simulink model "CASHEW_old"  (R2023a)
settings: Solver=ode23t  StartTime=0.0  StopTime=10.0  RelTol=1e-3
libraries: fl_lib x25, nesl_utility x9, SimscapeFluids_lib x7
settings Model: Creator=degoe  LastModifiedBy=cpoki

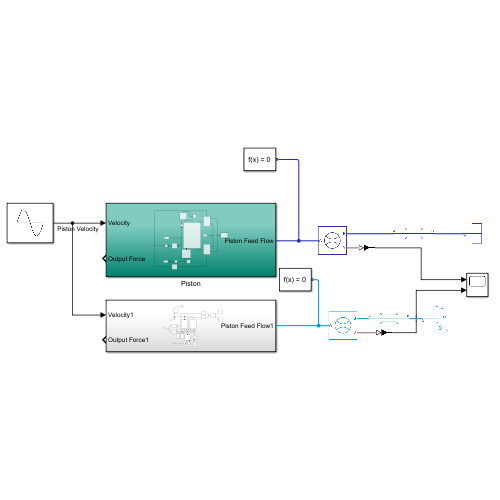
[thumbnail: Simulink's stored preview of the top-level diagram]
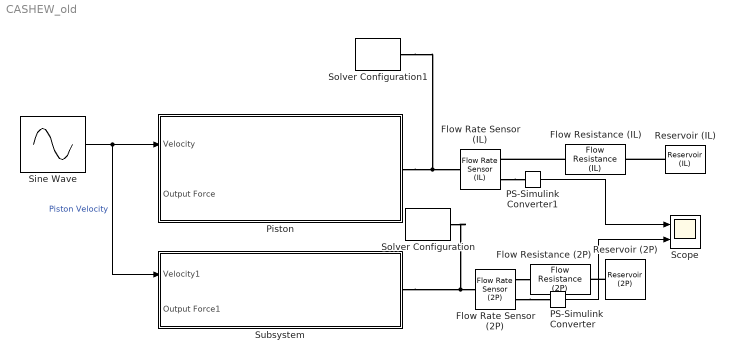
== system CASHEW_old ==
  Flow Rate Sensor (2P) : fl_lib/Two-Phase Fluid/Sensors/Flow Rate Sensor (2P)  mass_flow_measure=false  volumetric_flow_measure=true  energy_flow_measure=false
      settings: InternalSimscapePortConfiguration="{\"Bottom\":[],\"Left\":[{\"id\":\"A\",\"label\":\"A\",\"type\":\"foundation.two_phase_fluid.two_phase_fluid\"}],\"Right\":[{\"id\":\"B\",\"label\":\"B\",\"type\":\"foundation.two_phase_fluid.two_phase_fluid\"},{\"id\":\"V\",\"label\":\"V\",\"type\":\"output\"}],\"Top\":[]}"
  Flow Rate Sensor (IL) : fl_lib/Isothermal Liquid/Sensors/Flow Rate Sensor (IL)  sensor_type=foundation.enum.mass_volumetric_sensor.volumetric
      settings: InternalSimscapePortConfiguration="{\"Bottom\":[],\"Left\":[{\"id\":\"A\",\"label\":\"A\",\"type\":\"foundation.isothermal_liquid.isothermal_liquid\"}],\"Right\":[{\"id\":\"B\",\"label\":\"B\",\"type\":\"foundation.isothermal_liquid.isothermal_liquid\"},{\"id\":\"V\",\"label\":\"V\",\"type\":\"output\"}],\"Top\":[]}"
  Flow Resistance (2P) : fl_lib/Two-Phase Fluid/Elements/Flow Resistance (2P)  delta_p_nominal=0.001 MPa  mdot_nominal=0.1 kg/s  v_nominal=0 m^3/kg  area=0.01 m^2  laminar_fraction=1e-3
      settings: InternalSimscapePortConfiguration="{\"Bottom\":[],\"Left\":[{\"id\":\"A\",\"label\":\"A\",\"type\":\"foundation.two_phase_fluid.two_phase_fluid\"}],\"Right\":[{\"id\":\"B\",\"label\":\"B\",\"type\":\"foundation.two_phase_fluid.two_phase_fluid\"}],\"Top\":[]}"
  Flow Resistance (IL) : fl_lib/Isothermal Liquid/Elements/Flow Resistance (IL)  delta_p_nominal=0.001 MPa  mdot_nominal=0.1 kg/s  laminar_fraction=1e-3
      settings: InternalSimscapePortConfiguration="{\"Bottom\":[],\"Left\":[{\"id\":\"A\",\"label\":\"A\",\"type\":\"foundation.isothermal_liquid.isothermal_liquid\"}],\"Right\":[{\"id\":\"B\",\"label\":\"B\",\"type\":\"foundation.isothermal_liquid.isothermal_liquid\"}],\"Top\":[]}"
  PS-Simulink Converter : nesl_utility/PS-Simulink Converter  PhysicalDomain=network_engine_domain  SubClassName=ps_output  LeftPortType=input  RightPortType=output  PseudoPeriodic=off  Frequencies=[]  VectorFormat=inherit  Unit=inherit  AffineConversion=off
  PS-Simulink Converter1 : nesl_utility/PS-Simulink Converter  PhysicalDomain=network_engine_domain  SubClassName=ps_output  LeftPortType=input  RightPortType=output  PseudoPeriodic=off  Frequencies=[]  VectorFormat=inherit  Unit=inherit  AffineConversion=off
  Piston : Subsystem
      settings: PortSchema="{\"entries\":[{\"content\":{\"sides\":[{\"content\":{\"connectorIds\":[\"In1\",\"Out1\"]},\"type\":\"ConnectorPlacement.EquallySpacedRectSide\",\"uuid\":\"b8e78877-c290-4656-932c-79ee659867db\"},{\"content\":{\"connectorIds\":[\"RConn1\"],\"side\":\"RIGHT\"},\"type\":\"ConnectorPlacement.EquallySpacedRectSide\",\"uuid\":\"f3ba2138-776c-4b7b-9f4c-235aea75c0ff\"},{\"content\":{\"side\":\"TOP\"},\"type\":\"ConnectorPlacement.EquallySpacedRectSide\",\"uuid\":\"3b9ee6c7-725d-42d9-8cef-d327921b75c9\"}]},\"type\":\"ConnectorPlacement.EquallySpacedConnector\",\"uuid\":\"ca70cb4f-6465-4ac9-9ae0-4b805d4678c7\"}],\"packageUris\":[\"http://schema.mathworks.com/mf0/Connector/R2020b\"],\"version\":\"1.0\"}"
  Reservoir (2P) : fl_lib/Two-Phase Fluid/Elements/Reservoir (2P)  pressure_spec=foundation.enum.ReservoirPressureSpec2P.Atmospheric  reservoir_pressure=0.101325 MPa  reservoir_condensing_temperature=373.15 K  reservoir_evaporating_temperature=373.15 K  energy_spec=foundation.enum.ReservoirEnergySpec2P.Temperature  reservoir_temperature=293.15 K  reservoir_quality=0.5  reservoir_void_fraction=0.5  reservoir_enthalpy=1500 kJ/kg  reservoir_internal_energy=1500 kJ/kg  reservoir_subcooling=5 deltaK  reservoir_superheating=5 deltaK  area_A=0.01 m^2
  Reservoir (IL) : fl_lib/Isothermal Liquid/Elements/Reservoir (IL)  reservoir_type=foundation.enum.constant_controlled.constant  pressure_spec=foundation.enum.pressure_spec.atmospheric  reservoir_pressure=0.101325 MPa
  Scope : Scope  NumInputPorts=2
  Sine Wave : Sin  Amplitude=0.37233113  Frequency=0.7  SampleTime=0
  Solver Configuration : nesl_utility/Solver Configuration  PhysicalDomain=network_engine_domain  SubClassName=solver  LeftPortType=input  RightPortType=generic  Tones=[]  Harmonics=[]  SimulateNoise=off  Profile=off  UseLocalSampling=off  EnableSwitchedLinearOptims=on  FrequencyDomain=off  UseCCode=off  RelTol=0.001  AbsTol=0.001  MinStep=1e-09  ToWorkspace=off  RevertToSquareIcSolve=off  NumHomotopyIterations=100  PhasorMode=off  PhasorModeNumHarmonics=1  ConsistencySolver=NEWTON_XTOL_AFTER_FTOL  IndexReductionMethod=DerivativeReplacement  DoDC=off  ResidualTolerance=1e-09  ConsistencyTolSource=GLOBAL  ConsistencyAbsTol=0.001  ConsistencyRelTol=0.001  ConsistencyTolFactor=0.001  UseLocalSolver=off  LocalSolverChoice=NE_BACKWARD_EULER_ADVANCER  ResolveIndetEquations=on  FunctionEvalNumThread=1  LocalSolverSampleTime=0.001  DoFixedCost=off  MaxNonlinIter=3  MaxModeIter=2  ComputeImpulses=off  ImpulseIterations=2  LinearAlgebra=auto  LinearAlgebraNumThread=0  EquationFormulation=NE_TIME_EF  DelaysMemoryBudget=1024  AutomaticFiltering=on  FilteringTimeConstant=0.001  PartitionStorageMethod=AS_NEEDED  PartitionMemoryBudget=1024  PartitionMethod=ROBUST
  Solver Configuration1 : nesl_utility/Solver Configuration  PhysicalDomain=network_engine_domain  SubClassName=solver  LeftPortType=input  RightPortType=generic  Tones=[]  Harmonics=[]  SimulateNoise=off  Profile=off  UseLocalSampling=off  EnableSwitchedLinearOptims=on  FrequencyDomain=off  UseCCode=off  RelTol=0.001  AbsTol=0.001  MinStep=1e-09  ToWorkspace=off  RevertToSquareIcSolve=off  NumHomotopyIterations=100  PhasorMode=off  PhasorModeNumHarmonics=1  ConsistencySolver=NEWTON_XTOL_AFTER_FTOL  IndexReductionMethod=DerivativeReplacement  DoDC=off  ResidualTolerance=1e-09  ConsistencyTolSource=GLOBAL  ConsistencyAbsTol=0.001  ConsistencyRelTol=0.001  ConsistencyTolFactor=0.001  UseLocalSolver=off  LocalSolverChoice=NE_BACKWARD_EULER_ADVANCER  ResolveIndetEquations=on  FunctionEvalNumThread=1  LocalSolverSampleTime=0.001  DoFixedCost=off  MaxNonlinIter=3  MaxModeIter=2  ComputeImpulses=off  ImpulseIterations=2  LinearAlgebra=auto  LinearAlgebraNumThread=0  EquationFormulation=NE_TIME_EF  DelaysMemoryBudget=1024  AutomaticFiltering=on  FilteringTimeConstant=0.001  PartitionStorageMethod=AS_NEEDED  PartitionMemoryBudget=1024  PartitionMethod=ROBUST
  Subsystem : Subsystem
      settings: PortSchema="{\"entries\":[{\"content\":{\"sides\":[{\"content\":{\"connectorIds\":[\"In1\",\"Out1\"]},\"type\":\"ConnectorPlacement.EquallySpacedRectSide\",\"uuid\":\"3893c117-58f4-444a-acc3-3c8ad39863db\"},{\"content\":{\"connectorIds\":[\"RConn1\"],\"side\":\"RIGHT\"},\"type\":\"ConnectorPlacement.EquallySpacedRectSide\",\"uuid\":\"ce571c28-2e26-43fb-8d91-15cc15892142\"},{\"content\":{\"side\":\"TOP\"},\"type\":\"ConnectorPlacement.EquallySpacedRectSide\",\"uuid\":\"309e5996-fe42-4b39-b1f7-b2ffb0eab9ca\"}]},\"type\":\"ConnectorPlacement.EquallySpacedConnector\",\"uuid\":\"baf7f0f0-8da0-4833-91c3-445f9acfddc8\"}],\"packageUris\":[\"http://schema.mathworks.com/mf0/Connector/R2020b\"],\"version\":\"1.0\"}"
  wires:
  Sine Wave/1 -> Subsystem/1(Velocity1), Piston/1(Velocity)  "Piston Velocity"
  PS-Simulink Converter1/1 -> Scope/1
  PS-Simulink Converter/1 -> Scope/2
  connections:
  Subsystem/RConn1 -- Solver Configuration/RConn1 -- Flow Rate Sensor (2P)/LConn1
  Flow Rate Sensor (2P)/RConn1 -- Flow Resistance (2P)/LConn1
  Flow Rate Sensor (2P)/RConn2 -- PS-Simulink Converter/LConn1
  Piston/RConn1 -- Solver Configuration1/RConn1 -- Flow Rate Sensor (IL)/LConn1
  Flow Resistance (IL)/LConn1 -- Flow Rate Sensor (IL)/RConn1
  Flow Rate Sensor (IL)/RConn2 -- PS-Simulink Converter1/LConn1
  Reservoir (IL)/LConn1 -- Flow Resistance (IL)/RConn1
  Reservoir (2P)/LConn1 -- Flow Resistance (2P)/RConn1

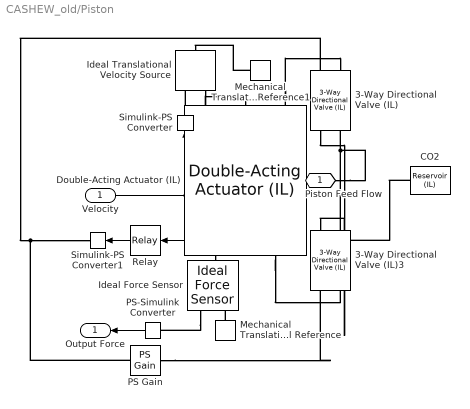
== system CASHEW_old/Piston ==
  Velocity : Inport
  3-Way Directional Valve (IL) : SimscapeFluids_lib/Isothermal Liquid/Valves & Orifices/Directional Control Valves/3-Way Directional Valve (IL)  open_orifices_pos=fluids.isothermal_liquid.valves_orifices.directional_control_valves.enum.DirectionalValveOpenOrifices3Way.PA  open_orifices_neg=fluids.isothermal_liquid.valves_orifices.directional_control_valves.enum.DirectionalValveOpenOrifices3Way.AT  area_spec=fluids.isothermal_liquid.valves_orifices.directional_control_valves.enum.directional_valve_area_spec.identical  valve_spec=fluids.isothermal_liquid.valves_orifices.directional_control_valves.enum.directional_valve_spec.linear  del_S_max=1 m  area_max=0.05 m^2  del_S_TLU=[0, .00125, .0025, .00375, .005] m  valve_area_TLU=[1e-10, 1e-05, 4e-05, 8e-05, .0001] m^2  del_S_vol_flow_TLU=[0, .00125, .0025, .00375, .005] m  p_diff_TLU=[-.1, .3, .5, .7] MPa  vol_flow_TLU=[-9.05e-10, 1.57e-09, 2.02e-09, 2.39e-09; -9.05e-05, .000157, .000202, .000239; -.000362, .000627, .00081, .000958; -.000724, .00125, .00162, .00192; -.000905, .00156, .002, .00239] m^3/s  area=inf m^2  area_leak=1e-15 m^2  Cd=0.7  Re_c=15000  smoothing_factor=0.01  pressure_recovery=false  S_max_PA=1 m  del_S_max_PA=0.005 m  area_max_PA=1e-4 m^2  del_S_TLU_PA=[0, .00125, .0025, .00375, .005] m  valve_area_TLU_PA=[1e-10, 1e-05, 4e-05, 8e-05, .0001] m^2  del_S_vol_flow_TLU_PA=[0, .00125, .0025, .00375, .005] m  p_diff_TLU_PA=[-.1, .3, .5, .7] MPa  vol_flow_TLU_PA=[-9.05e-10, 1.57e-09, 2.02e-09, 2.39e-09; -9.05e-05, .000157, .000202, .000239; -.000362, .000627, .00081, .000958; -.000724, .00125, .00162, .00192; -.000905, .00156, .002, .00239] m^3/s  S_max_AT=-1 m  del_S_max_AT=0.005 m  area_max_AT=1e-4 m^2  del_S_TLU_AT=[0, .00125, .0025, .00375, .005] m  valve_area_TLU_AT=[1e-10, 1e-05, 4e-05, 8e-05, .0001] m^2  del_S_vol_flow_TLU_AT=[0, .00125, .0025, .00375, .005] m  p_diff_TLU_AT=[-.1, .3, .5, .7] MPa  vol_flow_TLU_AT=[-9.05e-10, 1.57e-09, 2.02e-09, 2.39e-09; -9.05e-05, .000157, .000202, .000239; -.000362, .000627, .00081, .000958; -.000724, .00125, .00162, .00192; -.000905, .00156, .002, .00239] m^3/s  S_max_PT=4.5e-3 m  del_S_max_PT=0.005 m  area_max_PT=1e-4 m^2  del_S_TLU_PT=[0, .00125, .0025, .00375, .005] m  valve_area_TLU_PT=[1e-10, 1e-05, 4e-05, 8e-05, .0001] m^2  del_S_vol_flow_TLU_PT=[0, .00125, .0025, .00375, .005] m  p_diff_TLU_PT=[-.1, .3, .5, .7] MPa  vol_flow_TLU_PT=[-9.05e-10, 1.57e-09, 2.02e-09, 2.39e-09; -9.05e-05, .000157, .000202, .000239; -.000362, .000627, .00081, .000958; -.000724, .00125, .00162, .00192; -.000905, .00156, .002, .00239] m^3/s  enable_faults=simscape.enum.onoff.off  fault_type=fluids.enum.FaultSpool2Position.Positive  fault_trigger=foundation.enum.faultSpec.Temporal  fault_time=5 s
      settings: InternalSimscapePortConfiguration="{\"Bottom\":[{\"id\":\"P\",\"label\":\"P\",\"type\":\"foundation.isothermal_liquid.isothermal_liquid\"},{\"id\":\"T\",\"label\":\"T\",\"type\":\"foundation.isothermal_liquid.isothermal_liquid\"}],\"Left\":[{\"id\":\"S\",\"label\":\"S\",\"type\":\"input\"}],\"Right\":[],\"Top\":[{\"id\":\"A\",\"label\":\"A\",\"type\":\"foundation.isothermal_liquid.isothermal_liquid\"}]}"
  3-Way Directional Valve (IL)3 : SimscapeFluids_lib/Isothermal Liquid/Valves & Orifices/Directional Control Valves/3-Way Directional Valve (IL)  open_orifices_pos=fluids.isothermal_liquid.valves_orifices.directional_control_valves.enum.DirectionalValveOpenOrifices3Way.PA  open_orifices_neg=fluids.isothermal_liquid.valves_orifices.directional_control_valves.enum.DirectionalValveOpenOrifices3Way.AT  area_spec=fluids.isothermal_liquid.valves_orifices.directional_control_valves.enum.directional_valve_area_spec.identical  valve_spec=fluids.isothermal_liquid.valves_orifices.directional_control_valves.enum.directional_valve_spec.linear  del_S_max=1 m  area_max=0.05 m^2  del_S_TLU=[0, .00125, .0025, .00375, .005] m  valve_area_TLU=[1e-10, 1e-05, 4e-05, 8e-05, .0001] m^2  del_S_vol_flow_TLU=[0, .00125, .0025, .00375, .005] m  p_diff_TLU=[-.1, .3, .5, .7] MPa  vol_flow_TLU=[-9.05e-10, 1.57e-09, 2.02e-09, 2.39e-09; -9.05e-05, .000157, .000202, .000239; -.000362, .000627, .00081, .000958; -.000724, .00125, .00162, .00192; -.000905, .00156, .002, .00239] m^3/s  area=inf m^2  area_leak=1e-15 m^2  Cd=0.7  Re_c=15000  smoothing_factor=0.01  pressure_recovery=false  S_max_PA=1 m  del_S_max_PA=0.005 m  area_max_PA=1e-4 m^2  del_S_TLU_PA=[0, .00125, .0025, .00375, .005] m  valve_area_TLU_PA=[1e-10, 1e-05, 4e-05, 8e-05, .0001] m^2  del_S_vol_flow_TLU_PA=[0, .00125, .0025, .00375, .005] m  p_diff_TLU_PA=[-.1, .3, .5, .7] MPa  vol_flow_TLU_PA=[-9.05e-10, 1.57e-09, 2.02e-09, 2.39e-09; -9.05e-05, .000157, .000202, .000239; -.000362, .000627, .00081, .000958; -.000724, .00125, .00162, .00192; -.000905, .00156, .002, .00239] m^3/s  S_max_AT=-1 m  del_S_max_AT=0.005 m  area_max_AT=1e-4 m^2  del_S_TLU_AT=[0, .00125, .0025, .00375, .005] m  valve_area_TLU_AT=[1e-10, 1e-05, 4e-05, 8e-05, .0001] m^2  del_S_vol_flow_TLU_AT=[0, .00125, .0025, .00375, .005] m  p_diff_TLU_AT=[-.1, .3, .5, .7] MPa  vol_flow_TLU_AT=[-9.05e-10, 1.57e-09, 2.02e-09, 2.39e-09; -9.05e-05, .000157, .000202, .000239; -.000362, .000627, .00081, .000958; -.000724, .00125, .00162, .00192; -.000905, .00156, .002, .00239] m^3/s  S_max_PT=4.5e-3 m  del_S_max_PT=0.005 m  area_max_PT=1e-4 m^2  del_S_TLU_PT=[0, .00125, .0025, .00375, .005] m  valve_area_TLU_PT=[1e-10, 1e-05, 4e-05, 8e-05, .0001] m^2  del_S_vol_flow_TLU_PT=[0, .00125, .0025, .00375, .005] m  p_diff_TLU_PT=[-.1, .3, .5, .7] MPa  vol_flow_TLU_PT=[-9.05e-10, 1.57e-09, 2.02e-09, 2.39e-09; -9.05e-05, .000157, .000202, .000239; -.000362, .000627, .00081, .000958; -.000724, .00125, .00162, .00192; -.000905, .00156, .002, .00239] m^3/s  enable_faults=simscape.enum.onoff.off  fault_type=fluids.enum.FaultSpool2Position.Positive  fault_trigger=foundation.enum.faultSpec.Temporal  fault_time=5 s
      settings: InternalSimscapePortConfiguration="{\"Bottom\":[{\"id\":\"P\",\"label\":\"P\",\"type\":\"foundation.isothermal_liquid.isothermal_liquid\"},{\"id\":\"T\",\"label\":\"T\",\"type\":\"foundation.isothermal_liquid.isothermal_liquid\"}],\"Left\":[{\"id\":\"S\",\"label\":\"S\",\"type\":\"input\"}],\"Right\":[],\"Top\":[{\"id\":\"A\",\"label\":\"A\",\"type\":\"foundation.isothermal_liquid.isothermal_liquid\"}]}"
  CO2 : fl_lib/Isothermal Liquid/Elements/Reservoir (IL)  reservoir_type=foundation.enum.constant_controlled.constant  pressure_spec=foundation.enum.pressure_spec.atmospheric  reservoir_pressure=0.101325 MPa
  Double-Acting Actuator (IL) : SimscapeFluids_lib/Isothermal Liquid/Actuators/Double-Acting Actuator (IL)  mech_orientation=foundation.enum.MechOrientationTranslational.Positive  piston_area_A=piston_area m^2  piston_area_B=piston_area m^2  stroke=2000 m  dead_volume_A=1e-15 m^3  dead_volume_B=1e-15 m^3  pressure_spec=foundation.enum.pressure_spec.atmospheric  environment_pressure=0.101325 MPa  hardstop_model=simscape.enum.hardstop.smooth  stiff_coeff=1e10 N/m  damping_coeff=150 N*s/m  transition=0.1 mm  coeff_rest=0.7  v_tol=0.001 m/s  f_tol=0.001 N  cushion_A_spec=false  area_plunger_A=1e-4 m^2  length_plunger_A=1e-3 m  area_cushion_orifice_A=1e-6 m^2  area_leak_plunger_A=1e-7 m^2  p_crack_differential_A=0.01 MPa  press_max_differential_A=0.1 MPa  check_valve_area_max_A=1e-4 m^2  check_valve_area_leak_A=1e-10 m^2  smoothing_factor_A=0.01  cushion_B_spec=false  area_plunger_B=1e-4 m^2  length_plunger_B=1e-3 m  area_cushion_orifice_B=1e-6 m^2  area_leak_plunger_B=1e-7 m^2  p_crack_differential_B=0.01 MPa  press_max_differential_B=0.1 MPa  check_valve_area_max_B=1e-4 m^2  check_valve_area_leak_B=1e-10 m^2  smoothing_factor_B=0.01  friction_spec=false  breakaway_Coulomb_ratio=1.2  breakaway_velocity=0.1 m/s  preload_force=20 N  Coulomb_coeff=1e-6 N/Pa  viscous_coeff=100 N*s/m  leakage_spec=false  clearance=1e-4 m  piston_length=0.01 m  displacement_spec=foundation.enum.DisplacementSpec.Calculate  x0=6 m  dynamic_compressibility=false  p0_A=0.101325 MPa  p0_B=0.101325 MPa
      settings: InternalSimscapePortConfiguration="{\"Bottom\":[],\"Left\":[{\"id\":\"C\",\"label\":\"C\",\"type\":\"foundation.mechanical.translational.translational\"},{\"id\":\"A\",\"label\":\"A\",\"type\":\"foundation.isothermal_liquid.isothermal_liquid\"}],\"Right\":[{\"id\":\"p_out\",\"label\":\"p\",\"type\":\"output\"},{\"id\":\"R\",\"label\":\"R\",\"type\":\"foundation.mechanical.translational.translational\"},{\"id\":\"B\",\"label\":\"B\",\"type\":\"foundation.isothermal_liquid.isothermal_liquid\"}],\"Top\":[]}"
  Ideal Force Sensor : fl_lib/Mechanical/Mechanical Sensors/Ideal Force Sensor
  Ideal Translational Velocity Source : fl_lib/Mechanical/Mechanical Sources/Ideal Translational Velocity Source
  Mechanical Translational Reference : fl_lib/Mechanical/Translational Elements/Mechanical Translational Reference
  Mechanical Translational Reference1 : fl_lib/Mechanical/Translational Elements/Mechanical Translational Reference
  PS Gain : fl_lib/Physical Signals/Functions/PS Gain  gain=-1
  PS-Simulink Converter : nesl_utility/PS-Simulink Converter  PhysicalDomain=network_engine_domain  SubClassName=ps_output  LeftPortType=input  RightPortType=output  PseudoPeriodic=off  Frequencies=[]  VectorFormat=inherit  Unit=inherit  AffineConversion=off
  Relay : Relay  OnSwitchValue=0  OffSwitchValue=0  OffOutputValue=-1
  Simulink-PS Converter : nesl_utility/Simulink-PS Converter  PhysicalDomain=network_engine_domain  SubClassName=ps_input  LeftPortType=input  RightPortType=output  PseudoPeriodic=off  Frequencies=[]  NoiseDistribution=none  NoiseParameters=[]  Unit=m/s  AffineConversion=off  FilteringAndDerivatives=provide  SimscapeFilterOrder=1  InputFilterTimeConstant=0.001  UdotUserProvided=0
  Simulink-PS Converter1 : nesl_utility/Simulink-PS Converter  PhysicalDomain=network_engine_domain  SubClassName=ps_input  LeftPortType=input  RightPortType=output  PseudoPeriodic=off  Frequencies=[]  NoiseDistribution=none  NoiseParameters=[]  Unit=1  AffineConversion=off  FilteringAndDerivatives=provide  SimscapeFilterOrder=1  InputFilterTimeConstant=0.001  UdotUserProvided=0
  Piston Feed Flow : PMIOPort  Side=Right
  Output Force : Outport
  wires:
  Relay/1 -> Simulink-PS Converter1/1
  PS-Simulink Converter/1 -> Output Force/1
  Velocity/1 -> Simulink-PS Converter/1, Relay/1
  connections:
  PS Gain/LConn1 -- 3-Way Directional Valve (IL)/LConn1 -- Simulink-PS Converter1/RConn1
  Double-Acting Actuator (IL)/LConn1 -- Ideal Force Sensor/LConn1
  Simulink-PS Converter/RConn1 -- Ideal Translational Velocity Source/RConn1
  PS Gain/RConn1 -- 3-Way Directional Valve (IL)3/LConn1
  Double-Acting Actuator (IL)/LConn2 -- 3-Way Directional Valve (IL)3/LConn2
  Double-Acting Actuator (IL)/RConn3 -- 3-Way Directional Valve (IL)/LConn2
  3-Way Directional Valve (IL)3/RConn2 -- Piston Feed Flow/RConn1 -- 3-Way Directional Valve (IL)/RConn2
  3-Way Directional Valve (IL)/RConn1 -- CO2/LConn1 -- 3-Way Directional Valve (IL)3/RConn1
  Ideal Force Sensor/RConn2 -- PS-Simulink Converter/LConn1
  Mechanical Translational Reference/LConn1 -- Ideal Force Sensor/RConn1
  Mechanical Translational Reference1/LConn1 -- Ideal Translational Velocity Source/LConn1
  Ideal Translational Velocity Source/RConn2 -- Double-Acting Actuator (IL)/RConn2

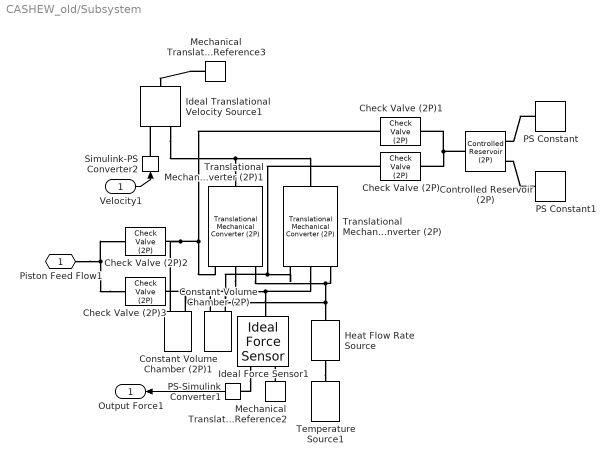
== system CASHEW_old/Subsystem ==
  Velocity1 : Inport
  Check Valve (2P){,1..3} (4 alike) : SimscapeFluids_lib/Two-Phase Fluid/Valves & Orifices/Directional Control Valves/Check Valve (2P)  opening_pressure_spec=fluids.two_phase_fluid.valves_orifices.enum.PressureControlSpec.Differential  p_crack_differential=0.01 MPa  p_crack_gauge=0.1 MPa  p_max_differential=0.1 MPa  p_max_gauge=0.2 MPa  mdot_nominal_max=0.1 kg/s  delta_p_nominal_max=0.001 MPa  energy_spec=foundation.enum.energy_spec.temperature  p_inlet=0.101325 MPa  T_inlet=293.15 K  x_inlet=0.5  alpha_inlet=0.5  h_inlet=1500 kJ/kg  u_inlet=1500 kJ/kg  area=0.01 m^2  mdot_leak_fraction=1e-6  smoothing_factor=0.01  B_lam=0.999  tau_x=0.1 s
      settings: InternalSimscapePortConfiguration="{\"Bottom\":[],\"Left\":[{\"id\":\"A\",\"label\":\"A\",\"type\":\"foundation.two_phase_fluid.two_phase_fluid\"}],\"Right\":[{\"id\":\"B\",\"label\":\"B\",\"type\":\"foundation.two_phase_fluid.two_phase_fluid\"}],\"Top\":[]}"
  Constant Volume Chamber (2P) : fl_lib/Two-Phase Fluid/Elements/Constant Volume Chamber (2P)  volume=0.001 m^3  num_ports=foundation.enum.num_ports.one  area_A=0.01 m^2  area_B=0.01 m^2  area_C=0.01 m^2  area_D=0.01 m^2  energy_spec=foundation.enum.energy_spec.temperature  p_init=0.101325 MPa  T_init=293.15 K  x_init=0.5  alpha_init=0.5  h_init=1500 kJ/kg  u_init=1500 kJ/kg  time_constant=0.1 s
      settings: InternalSimscapePortConfiguration="{\"Bottom\":[],\"Left\":[{\"id\":\"A\",\"label\":\"A\",\"type\":\"foundation.two_phase_fluid.two_phase_fluid\"},{\"id\":\"H\",\"label\":\"H\",\"type\":\"foundation.thermal.thermal\"}],\"Right\":[],\"Top\":[]}"
  Constant Volume Chamber (2P)1 : fl_lib/Two-Phase Fluid/Elements/Constant Volume Chamber (2P)  volume=0.001 m^3  num_ports=foundation.enum.num_ports.one  area_A=0.01 m^2  area_B=0.01 m^2  area_C=0.01 m^2  area_D=0.01 m^2  energy_spec=foundation.enum.energy_spec.temperature  p_init=0.101325 MPa  T_init=293.15 K  x_init=0.5  alpha_init=0.5  h_init=1500 kJ/kg  u_init=1500 kJ/kg  time_constant=0.1 s
      settings: InternalSimscapePortConfiguration="{\"Bottom\":[],\"Left\":[{\"id\":\"A\",\"label\":\"A\",\"type\":\"foundation.two_phase_fluid.two_phase_fluid\"},{\"id\":\"H\",\"label\":\"H\",\"type\":\"foundation.thermal.thermal\"}],\"Right\":[],\"Top\":[]}"
  Controlled Reservoir (2P) : fl_lib/Two-Phase Fluid/Elements/Controlled Reservoir (2P)  pressure_spec=foundation.enum.ControlledReservoirPressureSpec2P.Specified  energy_spec=foundation.enum.ControlledReservoirEnergySpec2P.LiquidTemperature  area_A=0.01 m^2  pressure_limit_spec=foundation.enum.PressureLimitSpec2P.Warn
      settings: InternalSimscapePortConfiguration="{\"Bottom\":[],\"Left\":[{\"id\":\"A\",\"label\":\"A\",\"type\":\"foundation.two_phase_fluid.two_phase_fluid\"}],\"Right\":[{\"id\":\"T\",\"label\":\"T\",\"type\":\"input\"},{\"id\":\"P\",\"label\":\"P\",\"type\":\"input\"}],\"Top\":[]}"
  Heat Flow Rate Source : fl_lib/Thermal/Thermal Sources/Heat Flow Rate Source  heat_flow=0 W
      settings: InternalSimscapePortConfiguration="{\"Bottom\":[],\"Left\":[{\"id\":\"B\",\"label\":\"B\",\"type\":\"foundation.thermal.thermal\"}],\"Right\":[{\"id\":\"A\",\"label\":\"A\",\"type\":\"foundation.thermal.thermal\"}],\"Top\":[]}"
  Ideal Force Sensor1 : fl_lib/Mechanical/Mechanical Sensors/Ideal Force Sensor
  Ideal Translational Velocity Source1 : fl_lib/Mechanical/Mechanical Sources/Ideal Translational Velocity Source
  Mechanical Translational Reference2 : fl_lib/Mechanical/Translational Elements/Mechanical Translational Reference
  Mechanical Translational Reference3 : fl_lib/Mechanical/Translational Elements/Mechanical Translational Reference
  PS Constant : fl_lib/Physical Signals/Sources/PS Constant  constant=101325 Pa
  PS Constant1 : fl_lib/Physical Signals/Sources/PS Constant  constant=293.15 K
  PS-Simulink Converter1 : nesl_utility/PS-Simulink Converter  PhysicalDomain=network_engine_domain  SubClassName=ps_output  LeftPortType=input  RightPortType=output  PseudoPeriodic=off  Frequencies=[]  VectorFormat=inherit  Unit=inherit  AffineConversion=off
  Simulink-PS Converter2 : nesl_utility/Simulink-PS Converter  PhysicalDomain=network_engine_domain  SubClassName=ps_input  LeftPortType=input  RightPortType=output  PseudoPeriodic=off  Frequencies=[]  NoiseDistribution=none  NoiseParameters=[]  Unit=m/s  AffineConversion=off  FilteringAndDerivatives=provide  SimscapeFilterOrder=1  InputFilterTimeConstant=0.001  UdotUserProvided=0
  Temperature Source1 : fl_lib/Thermal/Thermal Sources/Temperature Source  temperature=293.15 K
  Translational Mechanical Converter (2P) : fl_lib/Two-Phase Fluid/Elements/Translational Mechanical Converter (2P)  mech_orientation=foundation.enum.MechOrientationTranslational.Negative  displacement_spec=foundation.enum.DisplacementSpec.Calculate  length_init=0 m  interface_area=piston_area m^2  dead_volume=1e-5 m^3  area_A=0.01 m^2  pressure_spec=foundation.enum.pressure_spec.atmospheric  environment_pressure=0.101325 MPa  energy_spec=foundation.enum.energy_spec.temperature  p_init=0.101325 MPa  T_init=293.15 K  x_init=0.5  alpha_init=0.5  h_init=1500 kJ/kg  u_init=1500 kJ/kg  time_constant=0.1 s
      settings: InternalSimscapePortConfiguration="{\"Bottom\":[],\"Left\":[{\"id\":\"A\",\"label\":\"A\",\"type\":\"foundation.two_phase_fluid.two_phase_fluid\"},{\"id\":\"C\",\"label\":\"C\",\"type\":\"foundation.mechanical.translational.translational\"},{\"id\":\"H\",\"label\":\"H\",\"type\":\"foundation.thermal.thermal\"}],\"Right\":[{\"id\":\"R\",\"label\":\"R\",\"type\":\"foundation.mechanical.translational.translational\"}],\"Top\":[]}"
  Translational Mechanical Converter (2P)1 : fl_lib/Two-Phase Fluid/Elements/Translational Mechanical Converter (2P)  mech_orientation=foundation.enum.MechOrientationTranslational.Positive  displacement_spec=foundation.enum.DisplacementSpec.Calculate  length_init=0 m  interface_area=piston_area m^2  dead_volume=1e-5 m^3  area_A=0.01 m^2  pressure_spec=foundation.enum.pressure_spec.atmospheric  environment_pressure=0.101325 MPa  energy_spec=foundation.enum.energy_spec.temperature  p_init=0.101325 MPa  T_init=293.15 K  x_init=0.5  alpha_init=0.5  h_init=1500 kJ/kg  u_init=1500 kJ/kg  time_constant=0.1 s
      settings: InternalSimscapePortConfiguration="{\"Bottom\":[],\"Left\":[{\"id\":\"A\",\"label\":\"A\",\"type\":\"foundation.two_phase_fluid.two_phase_fluid\"},{\"id\":\"C\",\"label\":\"C\",\"type\":\"foundation.mechanical.translational.translational\"},{\"id\":\"H\",\"label\":\"H\",\"type\":\"foundation.thermal.thermal\"}],\"Right\":[{\"id\":\"R\",\"label\":\"R\",\"type\":\"foundation.mechanical.translational.translational\"}],\"Top\":[]}"
  Piston Feed Flow1 : PMIOPort  Side=Right
  Output Force1 : Outport
  wires:
  PS-Simulink Converter1/1 -> Output Force1/1
  Velocity1/1 -> Simulink-PS Converter2/1
  connections:
  Check Valve (2P)1/RConn1 -- Translational Mechanical Converter (2P)1/LConn1 -- Constant Volume Chamber (2P)1/LConn1 -- Check Valve (2P)2/LConn1
  Ideal Force Sensor1/LConn1 -- Translational Mechanical Converter (2P)/LConn2 -- Translational Mechanical Converter (2P)1/LConn2
  Check Valve (2P)1/LConn1 -- Controlled Reservoir (2P)/LConn1 -- Check Valve (2P)/LConn1
  Translational Mechanical Converter (2P)/LConn1 -- Check Valve (2P)/RConn1 -- Constant Volume Chamber (2P)/LConn1 -- Check Valve (2P)3/LConn1
  Check Valve (2P)3/RConn1 -- Piston Feed Flow1/RConn1 -- Check Valve (2P)2/RConn1
  Translational Mechanical Converter (2P)1/RConn1 -- Ideal Translational Velocity Source1/RConn2 -- Translational Mechanical Converter (2P)/RConn1
  Simulink-PS Converter2/RConn1 -- Ideal Translational Velocity Source1/RConn1
  Ideal Force Sensor1/RConn2 -- PS-Simulink Converter1/LConn1
  Mechanical Translational Reference3/LConn1 -- Ideal Translational Velocity Source1/LConn1
  Mechanical Translational Reference2/LConn1 -- Ideal Force Sensor1/RConn1
  PS Constant/RConn1 -- Controlled Reservoir (2P)/RConn2
  PS Constant1/RConn1 -- Controlled Reservoir (2P)/RConn1
  Translational Mechanical Converter (2P)1/LConn3 -- Translational Mechanical Converter (2P)/LConn3 -- Constant Volume Chamber (2P)1/LConn2 -- Constant Volume Chamber (2P)/LConn2 -- Heat Flow Rate Source/LConn1
  Heat Flow Rate Source/RConn1 -- Temperature Source1/LConn1
